simulink model "odometer2Wheels_soln"  (R2017a)
settings: Solver=VariableStepAuto  StartTime=0.0  StopTime=360  RelTol=1e-3
PreLoadFcn:
  | robotParameters;
  | ticksPerRot = 360;
values from neighbouring files (symbols this model uses):
  wheelR = 0.052    [robotParameters.m]
libraries: simulink x2
settings Model: Creator=sseshadr  LastModifiedBy=shiremat

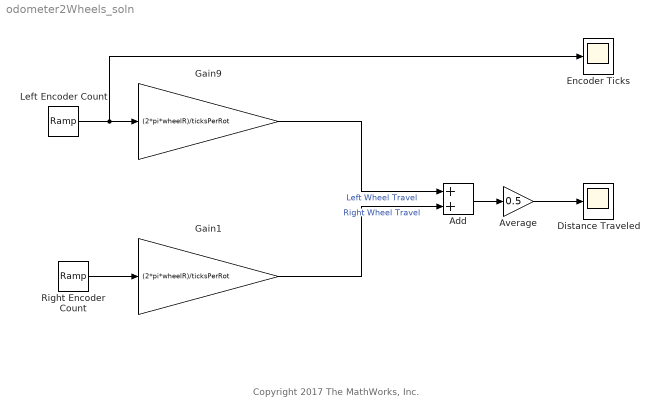
== system odometer2Wheels_soln ==
  note: Copyright 2017 The MathWorks, Inc.
  Add : Sum
  Average : Gain  Gain=0.5
  Distance Traveled : Scope
  Encoder Ticks : Scope
  Gain1 : Gain  Gain=(2*pi*wheelR)/ticksPerRot
  Gain9 : Gain  Gain=(2*pi*wheelR)/ticksPerRot
  Left Encoder Count : simulink/Sources/Ramp  slope=1  start=0  X0=0
  Right Encoder Count : simulink/Sources/Ramp  slope=-1  start=0  X0=0
  wires:
  Gain9/1 -> Add/1  "Left Wheel Travel"
  Right Encoder Count/1 -> Gain1/1
  Left Encoder Count/1 -> Gain9/1, Encoder Ticks/1
  Add/1 -> Average/1
  Average/1 -> Distance Traveled/1
  Gain1/1 -> Add/2  "Right Wheel Travel"
